simulink model "digital_tracking"  (R2017a)
settings: Solver=ode45  StartTime=0.0  StopTime=32  RelTol=1e-3  EnableMultiTasking=on
values from neighbouring files (symbols this model uses):
  A = [0 0 0 0 0 0 0 0 -9.30396437417 208.37461432 0 0 ... (36 elements, 6x6)]    [project_data.mat]
  B = [0  0; 0  0; 225.860837164  225.860837164; -49.0200587003  -49.0200587003; 0  0; -199954.688289  199954.688289]    [project_data.mat]
undefined symbols (not defined in the file or in its folder): C, gammaa, K1, K2, phia, T
libraries: simulink x1
settings Model: Creator=rjv  LastModifiedBy=kando
settings DataIOCC: LimitDataPoints=on  SaveFormat=Array
settings OptimizationCC: LifeSpan=inf
settings DebuggingCC: AllowSymbolicDim=off  SFUnexpectedBacktrackingDiag=warning  SFNoUnconditionalDefaultTransitionDiag=warning  SFExecutionAtInitializationDiag=none
settings HardwareCC: ProdBitPerPointer=32  ProdBitPerSizeT=32  ProdBitPerPtrDiffT=32  ProdLargestAtomicFloat=None  ProdIntDivRoundTo=Undefined  ProdEndianess=Unspecified  ProdWordSize=32  ProdHWDeviceType=32-bit Generic
settings ModelReferenceCC: PropagateSignalLabelsOutOfModel=off
settings GRTTargetCC: TargetLangStandard=C89/C90 (ANSI)  GeneratePreprocessorConditionals=Disable all
settings ConfigComp: CovMetricSettings=dw  CovHtmlReporting=on  CovSaveCumulativeToWorkspaceVar=on  CovSaveSingleToWorkspaceVar=on  CovExternalEMLEnable=off

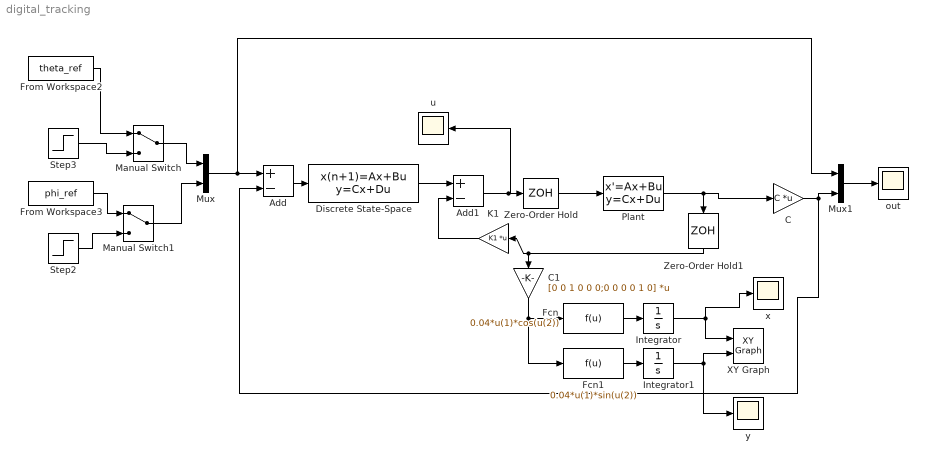
== system digital_tracking ==
  Add : Sum  Inputs=+-
  Add1 : Sum  Inputs=+-
  C : Gain  Gain=C  Multiplication=Matrix(K*u)
  C1 : Gain  Gain=[0 0 1 0 0 0;0 0 0 0 1 0]  Multiplication=Matrix(K*u)
  Discrete State-Space : DiscreteStateSpace  A=phia  B=gammaa  C=K2  D=0*K2*gammaa  X0=K2\(K1*[0;0;0;0;pi/4;0])  SampleTime=T
  Fcn : Fcn  Expr=0.04*u(1)*cos(u(2))
  Fcn1 : Fcn  Expr=0.04*u(1)*sin(u(2))
  From Workspace2 : FromWorkspace  VariableName=theta_ref  SampleTime=0.01  OutputAfterFinalValue=Holding final value
  From Workspace3 : FromWorkspace  VariableName=phi_ref  SampleTime=0.01  OutputAfterFinalValue=Holding final value
  Integrator : Integrator
  Integrator1 : Integrator
  K1 : Gain  Gain=K1  Multiplication=Matrix(K*u)
  Manual Switch : ManualSwitch
  Manual Switch1 : ManualSwitch
  Mux : Mux  Inputs=2
  Mux1 : Mux  Inputs=2
  Plant : StateSpace  A=A  B=B  C=eye(length(A))  D=zeros(length(A),min(size((B))))  X0=[0;0;0;0;pi/4;0]
  Step2 : Step  Time=0  Before=pi/4  After=pi/4+1  SampleTime=0
  Step3 : Step  Time=0  After=5  SampleTime=0
  XY Graph : simulink/Sinks/XY Graph  xmin=-1  xmax=1  ymin=-1  ymax=1  st=-1
  Zero-Order Hold : ZeroOrderHold  SampleTime=T
  Zero-Order Hold1 : ZeroOrderHold  SampleTime=T
  out : Scope
  u : Scope
  x : Scope
  y : Scope
  wires:
  Add1/1 -> Zero-Order Hold/1, u/1
  Discrete State-Space/1 -> Add1/1
  K1/1 -> Add1/2
  C/1 -> Add/2, Mux1/2
  Fcn/1 -> Integrator/1
  Fcn1/1 -> Integrator1/1
  Integrator/1 -> x/1, XY Graph/1
  Integrator1/1 -> y/1, XY Graph/2
  C1/1 -> Fcn/1, Fcn1/1
  Mux1/1 -> out/1
  Mux/1 -> Mux1/1, Add/1
  Step2/1 -> Manual Switch1/2
  From Workspace3/1 -> Manual Switch1/1
  Manual Switch1/1 -> Mux/2
  Manual Switch/1 -> Mux/1
  Step3/1 -> Manual Switch/2
  From Workspace2/1 -> Manual Switch/1
  Add/1 -> Discrete State-Space/1
  Zero-Order Hold/1 -> Plant/1
  Plant/1 -> Zero-Order Hold1/1, C/1
  Zero-Order Hold1/1 -> C1/1, K1/1
